simulink model "robotarm_part_both"  (R2018b)
settings: Solver=FixedStepAuto  StartTime=0.0  StopTime=options.T_train-options.dt  RelTol=1e-3  AbsTol=1e-6
undefined symbols (not defined in the file or in its folder): options
libraries: neural x132, simulink x4
(part 4 of 6)

== system robotarm_part_both/NN/Layer 3/Delays 1 ==
  "p{3}" : Inport  PortDimensions=30
      mask Display: e = 0.06;c1 = [120 230 180]/255;c2 = ([120 230 180]+0)/(256+128);c3 = ([120 230 180]+128)/(256+128);patch([0 1 1 0],[0 0 1 1],c1);patch([0 1 1 1-e 1-e 0+e],[0 0 1 1-e 0+e 0+e],c2);patch([0 0 1 1-e 0+e 0+e],[0 1 1 1-e 1-e 0+e],c3);plot([0 1 1 0 0],[0 0 1 1 0]);
  mux : Mux  Inputs=1
      mask Display: e = 0.06;c1 = [120 150 230]/255;c2 = ([120 150 230]+0)/383;c3 = ([120 150 230]+128)/383;patch([0 1 1 0],[0 0 1 1],c1);patch([0 1 1 1-e 1-e 0+e],[0 0 1 1-e 0+e 0+e],c2);patch([0 0 1 1-e 0+e 0+e],[0 1 1 1-e 1-e 0+e],c3);plot([0 1 1 0 0],[0 0 1 1 0]);disp('Mux')
  "pd{3,2}" : Outport
      mask Display: e = 0.06;c1 = [120 230 180]/255;c2 = ([120 230 180]+0)/(256+128);c3 = ([120 230 180]+128)/(256+128);patch([0 1 1 0],[0 0 1 1],c1);patch([0 1 1 1-e 1-e 0+e],[0 0 1 1-e 0+e 0+e],c2);patch([0 0 1 1-e 0+e 0+e],[0 1 1 1-e 1-e 0+e],c3);plot([0 1 1 0 0],[0 0 1 1 0]);
  wires:
  "p{3}"/1 -> mux/1
  mux/1 -> "pd{3,2}"/1

== system robotarm_part_both/NN/Layer 3/LW{3,2} ==
  "ad{3,2}" : Inport  PortDimensions=30
      mask Display: e = 0.06;c1 = [120 230 180]/255;c2 = ([120 230 180]+0)/(256+128);c3 = ([120 230 180]+128)/(256+128);patch([0 1 1 0],[0 0 1 1],c1);patch([0 1 1 1-e 1-e 0+e],[0 0 1 1-e 0+e 0+e],c2);patch([0 0 1 1-e 0+e 0+e],[0 1 1 1-e 1-e 0+e],c3);plot([0 1 1 0 0],[0 0 1 1 0]);
  "IW{3,2}(1,:)'" : Constant  Value=[0.176394547847553762043304459439241327345371246337890625;-0.1116456887869614333919088267066399566829204559326171875;0.58215121397970370775709625377203337848186492919921875;0.7323597745263732416987068063463084399700164794921875;0.283355295459314759920488313582609407603740692138671875;0.77930108203370540564947077655233442783355712890625;-0.28029976793160094050705311019555665552616119384765625;0.469261371288066830853580313487327657639980316162109375;0.292093450290357881105052229031571187078952789306640625;0.449281302149557693059733765039709396660327911376953125;0.386298724431223872155527487848303280770778656005859375;0.0105704306857183523427057281196539406664669513702392578125;-0.20177765854276685786317102611064910888671875;0.05511109655202676982366227775855804793536663055419921875;-0.5391171282818068011266632311162538826465606689453125;-0.41937710733039512689401817624457180500030517578125;-0.258060070180556488939060955090099014341831207275390625;-0.391205760480985542670850918511860072612762451171875;0.1540637115479316088251238170414580963551998138427734375;-0.372538014477659384926511165758711285889148712158203125;-0.7010359337987279726434053372940979897975921630859375;-0.3311213427238712814215659818728454411029815673828125;-0.07789499457458821940480930834382888861000537872314453125;-0.494423699379576142565184682098333723843097686767578125;-0.321664189878497486230202184742665849626064300537109375;-0.1524588096722032937169188926418428309261798858642578125;0.270977785627045497651721461807028390467166900634765625;-0.237034371203050320264793526803259737789630889892578125;-0.4681526216624172231917100361897610127925872802734375;-0.06115859490412589583030467110802419483661651611328125]
      mask Display: e = 0.06;c1 = [120 150 230]/255;c2 = ([120 150 230]+0)/383;c3 = ([120 150 230]+128)/383;patch([0 1 1 0],[0 0 1 1],c1);patch([0 1 1 1-e 1-e 0+e],[0 0 1 1-e 0+e 0+e],c2);patch([0 0 1 1-e 0+e 0+e],[0 1 1 1-e 1-e 0+e],c3);plot([0 1 1 0 0],[0 0 1 1 0]);disp('weights');
  Mux : Mux  Inputs=1
      mask Display: e = 0.06;c1 = [120 150 230]/255;c2 = ([120 150 230]+0)/383;c3 = ([120 150 230]+128)/383;patch([0 1 1 0],[0 0 1 1],c1);patch([0 1 1 1-e 1-e 0+e],[0 0 1 1-e 0+e 0+e],c2);patch([0 0 1 1-e 0+e 0+e],[0 1 1 1-e 1-e 0+e],c3);plot([0 1 1 0 0],[0 0 1 1 0]);disp('Mux');
  dotprod1 : neural/Weight Functions/dotprod
  "lz{3,2}" : Outport
      mask Display: e = 0.06;c1 = [120 230 180]/255;c2 = ([120 230 180]+0)/(256+128);c3 = ([120 230 180]+128)/(256+128);patch([0 1 1 0],[0 0 1 1],c1);patch([0 1 1 1-e 1-e 0+e],[0 0 1 1-e 0+e 0+e],c2);patch([0 0 1 1-e 0+e 0+e],[0 1 1 1-e 1-e 0+e],c3);plot([0 1 1 0 0],[0 0 1 1 0]);
  wires:
  "IW{3,2}(1,:)'"/1 -> dotprod1/1
  "ad{3,2}"/1 -> dotprod1/2
  dotprod1/1 -> Mux/1
  Mux/1 -> "lz{3,2}"/1

== system robotarm_part_both/NN_cex_1/Layer 1/Delays 1 ==
  "p{1}" : Inport  PortDimensions=10
      mask Display: e = 0.06;c1 = [120 230 180]/255;c2 = ([120 230 180]+0)/(256+128);c3 = ([120 230 180]+128)/(256+128);patch([0 1 1 0],[0 0 1 1],c1);patch([0 1 1 1-e 1-e 0+e],[0 0 1 1-e 0+e 0+e],c2);patch([0 0 1 1-e 0+e 0+e],[0 1 1 1-e 1-e 0+e],c3);plot([0 1 1 0 0],[0 0 1 1 0]);
  mux : Mux  Inputs=1
      mask Display: e = 0.06;c1 = [120 150 230]/255;c2 = ([120 150 230]+0)/383;c3 = ([120 150 230]+128)/383;patch([0 1 1 0],[0 0 1 1],c1);patch([0 1 1 1-e 1-e 0+e],[0 0 1 1-e 0+e 0+e],c2);patch([0 0 1 1-e 0+e 0+e],[0 1 1 1-e 1-e 0+e],c3);plot([0 1 1 0 0],[0 0 1 1 0]);disp('Mux')
  "pd{1,1}" : Outport
      mask Display: e = 0.06;c1 = [120 230 180]/255;c2 = ([120 230 180]+0)/(256+128);c3 = ([120 230 180]+128)/(256+128);patch([0 1 1 0],[0 0 1 1],c1);patch([0 1 1 1-e 1-e 0+e],[0 0 1 1-e 0+e 0+e],c2);patch([0 0 1 1-e 0+e 0+e],[0 1 1 1-e 1-e 0+e],c3);plot([0 1 1 0 0],[0 0 1 1 0]);
  wires:
  "p{1}"/1 -> mux/1
  mux/1 -> "pd{1,1}"/1

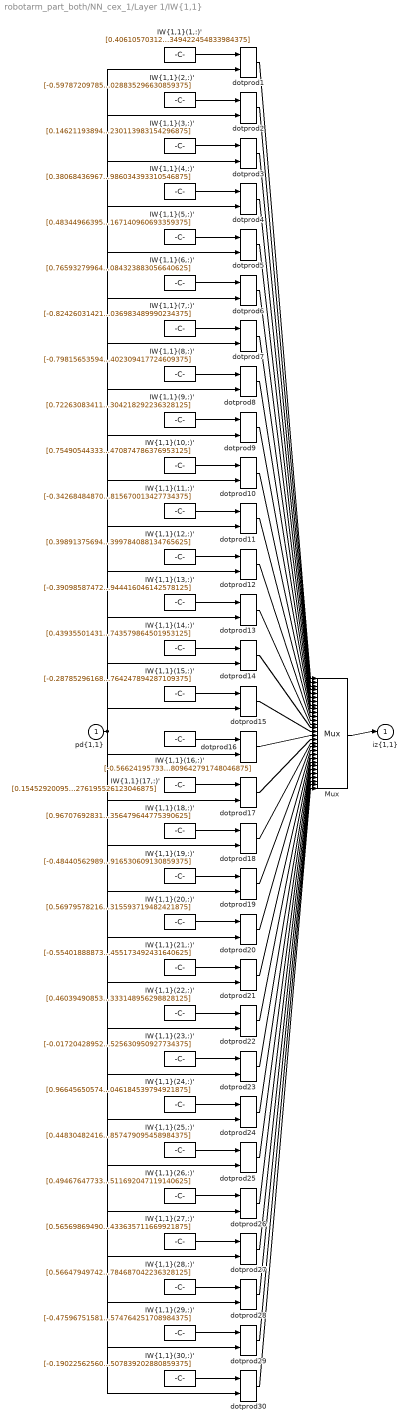
== system robotarm_part_both/NN_cex_1/Layer 1/IW{1,1} ==
  "pd{1,1}" : Inport  PortDimensions=10
      mask Display: e = 0.06;c1 = [120 230 180]/255;c2 = ([120 230 180]+0)/(256+128);c3 = ([120 230 180]+128)/(256+128);patch([0 1 1 0],[0 0 1 1],c1);patch([0 1 1 1-e 1-e 0+e],[0 0 1 1-e 0+e 0+e],c2);patch([0 0 1 1-e 0+e 0+e],[0 1 1 1-e 1-e 0+e],c3);plot([0 1 1 0 0],[0 0 1 1 0]);
  "IW{1,1}(1,:)'" : Constant  Value=[0.40610570312081251120872593673993833363056182861328125;-0.0618337729401200186796216939910664223134517669677734375;-0.027542948468563401009934210605933913029730319976806640625;-0.74658296364276865997311460887431167066097259521484375;0.0647152481491918563083487470066756941378116607666015625;0.532009309863485935210292154806666076183319091796875;-0.051795183452861430495328676215649466030299663543701171875;1.16180416143057296807228340185247361660003662109375;0.403930434889277767407378405550844036042690277099609375;-0.70819180118117885935902222627191804349422454833984375]
      mask Display: e = 0.06;c1 = [120 150 230]/255;c2 = ([120 150 230]+0)/383;c3 = ([120 150 230]+128)/383;patch([0 1 1 0],[0 0 1 1],c1);patch([0 1 1 1-e 1-e 0+e],[0 0 1 1-e 0+e 0+e],c2);patch([0 0 1 1-e 0+e 0+e],[0 1 1 1-e 1-e 0+e],c3);plot([0 1 1 0 0],[0 0 1 1 0]);disp('Weights');
  "IW{1,1}(10,:)'" : Constant  Value=[0.754905443337720694074732818990014493465423583984375;-0.2307145756276104131554660625624819658696651458740234375;-0.058374557330017916301212466123615740798413753509521484375;0.80634010994632199231801905625616200268268585205078125;-0.387179161003805616392270394499064423143863677978515625;0.4883646797805132333536448641098104417324066162109375;0.9334065215820845917704673411208204925060272216796875;-0.68294902726114614655017476252396591007709503173828125;0.57946714263174925463317777030169963836669921875;-0.384973810509336378249400922868517227470874786376953125]
      mask Display: e = 0.06;c1 = [120 150 230]/255;c2 = ([120 150 230]+0)/383;c3 = ([120 150 230]+128)/383;patch([0 1 1 0],[0 0 1 1],c1);patch([0 1 1 1-e 1-e 0+e],[0 0 1 1-e 0+e 0+e],c2);patch([0 0 1 1-e 0+e 0+e],[0 1 1 1-e 1-e 0+e],c3);plot([0 1 1 0 0],[0 0 1 1 0]);disp('Weights');
  "IW{1,1}(11,:)'" : Constant  Value=[-0.342684848708500300329404808508115820586681365966796875;-0.4011699929023067046074402242084033787250518798828125;1.0598889739814121302430294235819019377231597900390625;-0.2566824900326813985174112531240098178386688232421875;0.286617566677122737051064405022771097719669342041015625;0.437452894939382719297071844266611151397228240966796875;-0.83506440735054210389165518790832720696926116943359375;0.281658478227369057922402362237335182726383209228515625;0.47340709091096166982737258877023123204708099365234375;0.98784426306218531266267746104858815670013427734375]
      mask Display: e = 0.06;c1 = [120 150 230]/255;c2 = ([120 150 230]+0)/383;c3 = ([120 150 230]+128)/383;patch([0 1 1 0],[0 0 1 1],c1);patch([0 1 1 1-e 1-e 0+e],[0 0 1 1-e 0+e 0+e],c2);patch([0 0 1 1-e 0+e 0+e],[0 1 1 1-e 1-e 0+e],c3);plot([0 1 1 0 0],[0 0 1 1 0]);disp('Weights');
  "IW{1,1}(12,:)'" : Constant  Value=[0.398913756949194342471542995554045774042606353759765625;-1.0219642473780263802751733237528242170810699462890625;0.66452831996743022546780821357970125973224639892578125;0.7230875011438542276920315998722799122333526611328125;0.06718552543198720583550453966381610371172428131103515625;0.25328258897489164258587379663367755711078643798828125;0.04377790583161665638467496819430380128324031829833984375;0.2465544725107126355911901782747008837759494781494140625;0.380746784031783802593196242014528252184391021728515625;0.698639278926427298443968538776971399784088134765625]
      mask Display: e = 0.06;c1 = [120 150 230]/255;c2 = ([120 150 230]+0)/383;c3 = ([120 150 230]+128)/383;patch([0 1 1 0],[0 0 1 1],c1);patch([0 1 1 1-e 1-e 0+e],[0 0 1 1-e 0+e 0+e],c2);patch([0 0 1 1-e 0+e 0+e],[0 1 1 1-e 1-e 0+e],c3);plot([0 1 1 0 0],[0 0 1 1 0]);disp('Weights');
  "IW{1,1}(13,:)'" : Constant  Value=[-0.390985874725247761762858544898335821926593780517578125;0.68715563779107657893518990022130310535430908203125;-0.05459024117889653415769402045043534599244594573974609375;0.493818674941325530536317955920821987092494964599609375;0.93328497180974079316939651107531972229480743408203125;-0.04136663725988042050740745025905198417603969573974609375;0.51698619349367913589077261349302716553211212158203125;-0.2237583707189104986756689186222502030432224273681640625;0.63723107769787101783975913349422626197338104248046875;-0.888813604233327669845721175079233944416046142578125]
      mask Display: e = 0.06;c1 = [120 150 230]/255;c2 = ([120 150 230]+0)/383;c3 = ([120 150 230]+128)/383;patch([0 1 1 0],[0 0 1 1],c1);patch([0 1 1 1-e 1-e 0+e],[0 0 1 1-e 0+e 0+e],c2);patch([0 0 1 1-e 0+e 0+e],[0 1 1 1-e 1-e 0+e],c3);plot([0 1 1 0 0],[0 0 1 1 0]);disp('Weights');
  "IW{1,1}(14,:)'" : Constant  Value=[0.439355014317911740651112495470442809164524078369140625;-0.6120670869240980582759448225260712206363677978515625;-0.80865955894022889527406050547142513096332550048828125;0.371840320627411846654553073676652275025844573974609375;-0.94104647756993109464218605353380553424358367919921875;1.0656100492619675623728880964335985481739044189453125;0.215787684182779881947311650947085581719875335693359375;0.305366971574978440795433698440319858491420745849609375;-0.03747921878648863280858449797960929572582244873046875;0.114143621883545709483342989187804050743579864501953125]
      mask Display: e = 0.06;c1 = [120 150 230]/255;c2 = ([120 150 230]+0)/383;c3 = ([120 150 230]+128)/383;patch([0 1 1 0],[0 0 1 1],c1);patch([0 1 1 1-e 1-e 0+e],[0 0 1 1-e 0+e 0+e],c2);patch([0 0 1 1-e 0+e 0+e],[0 1 1 1-e 1-e 0+e],c3);plot([0 1 1 0 0],[0 0 1 1 0]);disp('Weights');
  "IW{1,1}(15,:)'" : Constant  Value=[-0.287852961686321240364350160234607756137847900390625;0.193811697275944105900435943112825043499469757080078125;-0.8410307478423624250041257255361415445804595947265625;0.84437904998481816409849898263928480446338653564453125;0.29952993297291474750210227284696884453296661376953125;0.27291419885216672280847660658764652907848358154296875;0.6419725776834723784958214309881441295146942138671875;-0.10748546258155665389377730889464146457612514495849609375;-0.478464668092987377434610607451759278774261474609375;-0.6291180402851974662326028919778764247894287109375]
      mask Display: e = 0.06;c1 = [120 150 230]/255;c2 = ([120 150 230]+0)/383;c3 = ([120 150 230]+128)/383;patch([0 1 1 0],[0 0 1 1],c1);patch([0 1 1 1-e 1-e 0+e],[0 0 1 1-e 0+e 0+e],c2);patch([0 0 1 1-e 0+e 0+e],[0 1 1 1-e 1-e 0+e],c3);plot([0 1 1 0 0],[0 0 1 1 0]);disp('Weights');
  "IW{1,1}(16,:)'" : Constant  Value=[-0.5662419573309234177571624968550167977809906005859375;0.504981057654423803882082211202941834926605224609375;-1.1343989356561134940193369402550160884857177734375;-0.075054956664876215644000012616743333637714385986328125;-0.85555149227211002571635845015407539904117584228515625;-0.189969480968393444886288534689811058342456817626953125;0.257703553768643456312048556355875916779041290283203125;-0.114101898538623292012061938294209539890289306640625;-0.01034982455533548471870997076393905445002019405364990234375;-0.03712863475843779237361985678944620303809642791748046875]
      mask Display: e = 0.06;c1 = [120 150 230]/255;c2 = ([120 150 230]+0)/383;c3 = ([120 150 230]+128)/383;patch([0 1 1 0],[0 0 1 1],c1);patch([0 1 1 1-e 1-e 0+e],[0 0 1 1-e 0+e 0+e],c2);patch([0 0 1 1-e 0+e 0+e],[0 1 1 1-e 1-e 0+e],c3);plot([0 1 1 0 0],[0 0 1 1 0]);disp('Weights');
  "IW{1,1}(17,:)'" : Constant  Value=[0.154529200951685208309527297387830913066864013671875;0.48354369097717586623019769831444136798381805419921875;0.692335704444002164592575354618020355701446533203125;0.33065881691269505271435491522424854338169097900390625;0.700715460652138855124348992831073701381683349609375;0.9392393355523533937656566195073537528514862060546875;-0.83768647200012946729685836544376797974109649658203125;-0.278233473644368178856467466175672598183155059814453125;0.375486157959734168088061778689734637737274169921875;0.11365059515114765698040599772866698913276195526123046875]
      mask Display: e = 0.06;c1 = [120 150 230]/255;c2 = ([120 150 230]+0)/383;c3 = ([120 150 230]+128)/383;patch([0 1 1 0],[0 0 1 1],c1);patch([0 1 1 1-e 1-e 0+e],[0 0 1 1-e 0+e 0+e],c2);patch([0 0 1 1-e 0+e 0+e],[0 1 1 1-e 1-e 0+e],c3);plot([0 1 1 0 0],[0 0 1 1 0]);disp('Weights');
  "IW{1,1}(18,:)'" : Constant  Value=[0.967076928319382300713868971797637641429901123046875;-0.66164947528674133980786109532346017658710479736328125;-0.3141703919957035129328914990765042603015899658203125;-0.93982557986142711836663465874153189361095428466796875;-0.5448594698446898032528906696825288236141204833984375;0.1274965495680859539628926313525880686938762664794921875;0.403484102726418936146757232563686557114124298095703125;-0.450081409216426531205712535665952600538730621337890625;0.404013712675034331045509361501899547874927520751953125;0.69614128919235407355614597690873779356479644775390625]
      mask Display: e = 0.06;c1 = [120 150 230]/255;c2 = ([120 150 230]+0)/383;c3 = ([120 150 230]+128)/383;patch([0 1 1 0],[0 0 1 1],c1);patch([0 1 1 1-e 1-e 0+e],[0 0 1 1-e 0+e 0+e],c2);patch([0 0 1 1-e 0+e 0+e],[0 1 1 1-e 1-e 0+e],c3);plot([0 1 1 0 0],[0 0 1 1 0]);disp('Weights');
  "IW{1,1}(19,:)'" : Constant  Value=[-0.484405629893030875710024929503560997545719146728515625;0.77945971793746637867883464423357509076595306396484375;-0.278649568567306105126846205166657455265522003173828125;0.49799572768193989258378451268072240054607391357421875;-0.388289522122739760856546809009159915149211883544921875;0.162724212432617532098078072522184811532497406005859375;0.764539980173248867600932499044574797153472900390625;-0.6912157507333909212121625387226231396198272705078125;-0.9166608172565313683577414849423803389072418212890625;-0.7061016716226686806834322851500473916530609130859375]
      mask Display: e = 0.06;c1 = [120 150 230]/255;c2 = ([120 150 230]+0)/383;c3 = ([120 150 230]+128)/383;patch([0 1 1 0],[0 0 1 1],c1);patch([0 1 1 1-e 1-e 0+e],[0 0 1 1-e 0+e 0+e],c2);patch([0 0 1 1-e 0+e 0+e],[0 1 1 1-e 1-e 0+e],c3);plot([0 1 1 0 0],[0 0 1 1 0]);disp('Weights');
  "IW{1,1}(2,:)'" : Constant  Value=[-0.5978720978507292560522046187543310225009918212890625;-0.451225889460342977077544901476358063519001007080078125;0.73115114985429396909921706537716090679168701171875;-0.33177832418549713100475173632730729877948760986328125;0.5656634448348001331652312728692777454853057861328125;0.203845531538278501582084345500334165990352630615234375;0.60328541488133613501787522181984968483448028564453125;-0.295759245605732079553717994713224470615386962890625;-0.863527859816612508581101792515255510807037353515625;-0.8686108953587632353077196967205964028835296630859375]
      mask Display: e = 0.06;c1 = [120 150 230]/255;c2 = ([120 150 230]+0)/383;c3 = ([120 150 230]+128)/383;patch([0 1 1 0],[0 0 1 1],c1);patch([0 1 1 1-e 1-e 0+e],[0 0 1 1-e 0+e 0+e],c2);patch([0 0 1 1-e 0+e 0+e],[0 1 1 1-e 1-e 0+e],c3);plot([0 1 1 0 0],[0 0 1 1 0]);disp('Weights');
  "IW{1,1}(20,:)'" : Constant  Value=[0.569795782163188935243169908062554895877838134765625;-0.175366068818801290607467535664909519255161285400390625;0.299468569242130888685693435036228038370609283447265625;0.00013019514896176246319947633622859939350746572017669677734375;-0.913508827616769547574904208886437118053436279296875;1.2317060303614313365727639393298886716365814208984375;-0.310041832148403584401563648498267866671085357666015625;-0.68644604330826031191037372991559095680713653564453125;-0.02734988959488722504165281179666635580360889434814453125;-0.1646195679784154541902552182364161126315593719482421875]
      mask Display: e = 0.06;c1 = [120 150 230]/255;c2 = ([120 150 230]+0)/383;c3 = ([120 150 230]+128)/383;patch([0 1 1 0],[0 0 1 1],c1);patch([0 1 1 1-e 1-e 0+e],[0 0 1 1-e 0+e 0+e],c2);patch([0 0 1 1-e 0+e 0+e],[0 1 1 1-e 1-e 0+e],c3);plot([0 1 1 0 0],[0 0 1 1 0]);disp('Weights');
  "IW{1,1}(21,:)'" : Constant  Value=[-0.554018888738172510244339719065465033054351806640625;-0.428769524213964914327590349785168655216693878173828125;-0.0800834615707680941287804898820468224585056304931640625;-0.8169714872980133879565300958347506821155548095703125;-0.6459854934693691763669676220160908997058868408203125;0.58988824050972965551409288309514522552490234375;0.2646341908830576183930816114298067986965179443359375;-0.68226497917992612318727196907275356352329254150390625;0.389913364883176460917724170940346084535121917724609375;0.671389074260846374642142109223641455173492431640625]
      mask Display: e = 0.06;c1 = [120 150 230]/255;c2 = ([120 150 230]+0)/383;c3 = ([120 150 230]+128)/383;patch([0 1 1 0],[0 0 1 1],c1);patch([0 1 1 1-e 1-e 0+e],[0 0 1 1-e 0+e 0+e],c2);patch([0 0 1 1-e 0+e 0+e],[0 1 1 1-e 1-e 0+e],c3);plot([0 1 1 0 0],[0 0 1 1 0]);disp('Weights');
  "IW{1,1}(22,:)'" : Constant  Value=[0.460394908538499125771892295233556069433689117431640625;0.69299410430707297781083298104931600391864776611328125;-0.58147459969207215824127388259512372314929962158203125;-0.474008418395088726438046933253644965589046478271484375;-0.19586296063152819346697697255876846611499786376953125;-0.5774582392745102321640615627984516322612762451171875;0.915756888185493611587162376963533461093902587890625;-0.844006379670238171541996052837930619716644287109375;-0.62517377429491582940812577362521551549434661865234375;-0.394218307905169595972694196461816318333148956298828125]
      mask Display: e = 0.06;c1 = [120 150 230]/255;c2 = ([120 150 230]+0)/383;c3 = ([120 150 230]+128)/383;patch([0 1 1 0],[0 0 1 1],c1);patch([0 1 1 1-e 1-e 0+e],[0 0 1 1-e 0+e 0+e],c2);patch([0 0 1 1-e 0+e 0+e],[0 1 1 1-e 1-e 0+e],c3);plot([0 1 1 0 0],[0 0 1 1 0]);disp('Weights');
  "IW{1,1}(23,:)'" : Constant  Value=[-0.01720428952464754523976608879820560105144977569580078125;0.0915619286382170771698696398743777535855770111083984375;-0.216310552483802209788876780294231139123439788818359375;0.683699817299082912569474501651711761951446533203125;0.55572107062446374214914612821303308010101318359375;-0.38831201307937046607321462943218648433685302734375;0.74460998939169098509438526889425702393054962158203125;-0.412168552568078883080460173005121760070323944091796875;0.296429067542405111357339819733169861137866973876953125;-0.903105169254780459908715783967636525630950927734375]
      mask Display: e = 0.06;c1 = [120 150 230]/255;c2 = ([120 150 230]+0)/383;c3 = ([120 150 230]+128)/383;patch([0 1 1 0],[0 0 1 1],c1);patch([0 1 1 1-e 1-e 0+e],[0 0 1 1-e 0+e 0+e],c2);patch([0 0 1 1-e 0+e 0+e],[0 1 1 1-e 1-e 0+e],c3);plot([0 1 1 0 0],[0 0 1 1 0]);disp('Weights');
  "IW{1,1}(24,:)'" : Constant  Value=[0.9664565057440073214678477597772143781185150146484375;0.08297129843086743783420189402022515423595905303955078125;-0.782415106607832644414202150073833763599395751953125;-0.62027706726544362680897393147461116313934326171875;0.7418119761811379220262097078375518321990966796875;-0.7912576799074060307503941658069379627704620361328125;0.15814280110847656057870835866197012364864349365234375;-0.47819226762323463475468088290654122829437255859375;0.44516983178018654232488415800617076456546783447265625;-0.1378403995316616892363725810355390422046184539794921875]
      mask Display: e = 0.06;c1 = [120 150 230]/255;c2 = ([120 150 230]+0)/383;c3 = ([120 150 230]+128)/383;patch([0 1 1 0],[0 0 1 1],c1);patch([0 1 1 1-e 1-e 0+e],[0 0 1 1-e 0+e 0+e],c2);patch([0 0 1 1-e 0+e 0+e],[0 1 1 1-e 1-e 0+e],c3);plot([0 1 1 0 0],[0 0 1 1 0]);disp('Weights');
  "IW{1,1}(25,:)'" : Constant  Value=[0.448304824162995718683788481939700432121753692626953125;-0.441083545672387666858327293084585107862949371337890625;-0.7086421050067974736208498143241740763187408447265625;0.805571336795230852345639505074359476566314697265625;0.7757330590206288345456187016679905354976654052734375;-0.258695728383482370649204540313803590834140777587890625;-0.40794372310651982882490074189263395965099334716796875;0.264501362790562855042963974483427591621875762939453125;0.56836095891894611309425044964882545173168182373046875;0.94902066957128194957249434082768857479095458984375]
      mask Display: e = 0.06;c1 = [120 150 230]/255;c2 = ([120 150 230]+0)/383;c3 = ([120 150 230]+128)/383;patch([0 1 1 0],[0 0 1 1],c1);patch([0 1 1 1-e 1-e 0+e],[0 0 1 1-e 0+e 0+e],c2);patch([0 0 1 1-e 0+e 0+e],[0 1 1 1-e 1-e 0+e],c3);plot([0 1 1 0 0],[0 0 1 1 0]);disp('Weights');
  "IW{1,1}(26,:)'" : Constant  Value=[0.494676477332296193889504820617730729281902313232421875;-0.51418734519718201081417419118224643170833587646484375;-0.53269214219483107530805909846094436943531036376953125;-0.326399857319428277069306432167650200426578521728515625;-0.641083256409577639800545512116514146327972412109375;-0.661372013967330030226321468944661319255828857421875;-0.51378225686084999512814874833566136658191680908203125;-0.7031859535346625111884577563614584505558013916015625;0.71167339493647296944089930548216216266155242919921875;-0.253121486450810895263430211343802511692047119140625]
      mask Display: e = 0.06;c1 = [120 150 230]/255;c2 = ([120 150 230]+0)/383;c3 = ([120 150 230]+128)/383;patch([0 1 1 0],[0 0 1 1],c1);patch([0 1 1 1-e 1-e 0+e],[0 0 1 1-e 0+e 0+e],c2);patch([0 0 1 1-e 0+e 0+e],[0 1 1 1-e 1-e 0+e],c3);plot([0 1 1 0 0],[0 0 1 1 0]);disp('Weights');
  "IW{1,1}(27,:)'" : Constant  Value=[0.56569869490757884733511673402972519397735595703125;0.55932485469986747972370721981860697269439697265625;0.757553169851645780141780051053501665592193603515625;0.445739884859973678477018665944342501461505889892578125;-0.052810541890100599904389611083388444967567920684814453125;-0.5124647759251439449457166119827888906002044677734375;0.1453672125440539086849156547032180242240428924560546875;0.5844524834818864977847852060222066938877105712890625;0.301678561512196796723372926862793974578380584716796875;0.67239156025882074185773262797738425433635711669921875]
      mask Display: e = 0.06;c1 = [120 150 230]/255;c2 = ([120 150 230]+0)/383;c3 = ([120 150 230]+128)/383;patch([0 1 1 0],[0 0 1 1],c1);patch([0 1 1 1-e 1-e 0+e],[0 0 1 1-e 0+e 0+e],c2);patch([0 0 1 1-e 0+e 0+e],[0 1 1 1-e 1-e 0+e],c3);plot([0 1 1 0 0],[0 0 1 1 0]);disp('Weights');
  "IW{1,1}(28,:)'" : Constant  Value=[0.56647949742772751857700086475233547389507293701171875;-0.6072031078302975171112620955682359635829925537109375;-0.0252895405359683279888916018762756721116602420806884765625;-0.59420130639994450660879010683856904506683349609375;-0.8370146046590443145163362714811228215694427490234375;-0.2168133856068210629786108256666921079158782958984375;-0.0278184788230993497448739759647651226259768009185791015625;0.170700644385492206200893861023359932005405426025390625;-0.89753992568694818121599610094563104212284088134765625;-0.88615362909724126883048711533774621784687042236328125]
      mask Display: e = 0.06;c1 = [120 150 230]/255;c2 = ([120 150 230]+0)/383;c3 = ([120 150 230]+128)/383;patch([0 1 1 0],[0 0 1 1],c1);patch([0 1 1 1-e 1-e 0+e],[0 0 1 1-e 0+e 0+e],c2);patch([0 0 1 1-e 0+e 0+e],[0 1 1 1-e 1-e 0+e],c3);plot([0 1 1 0 0],[0 0 1 1 0]);disp('Weights');
  "IW{1,1}(29,:)'" : Constant  Value=[-0.47596751581870855307698775504832156002521514892578125;0.61043374535515082524028684929362498223781585693359375;0.6728816456322224137664989029872231185436248779296875;0.486894561880593490510449328212416730821132659912109375;0.61933355086790087273840299531002528965473175048828125;-0.457033928935499600409997356109670363366603851318359375;-0.66696973339012910475531725751352496445178985595703125;-0.5293927524224042446832072528195567429065704345703125;0.0993688407071657009428378160009742714464664459228515625;0.8282155411331133532115700290887616574764251708984375]
      mask Display: e = 0.06;c1 = [120 150 230]/255;c2 = ([120 150 230]+0)/383;c3 = ([120 150 230]+128)/383;patch([0 1 1 0],[0 0 1 1],c1);patch([0 1 1 1-e 1-e 0+e],[0 0 1 1-e 0+e 0+e],c2);patch([0 0 1 1-e 0+e 0+e],[0 1 1 1-e 1-e 0+e],c3);plot([0 1 1 0 0],[0 0 1 1 0]);disp('Weights');
  "IW{1,1}(3,:)'" : Constant  Value=[0.1462119389481443543221672598519944585859775543212890625;0.5409826763721661269102014557574875652790069580078125;-0.5796650085556314113688358702347613871097564697265625;-0.30474880936511306028791068456484936177730560302734375;0.564453778928731164654664098634384572505950927734375;-0.81205952454796881401222208296530880033969879150390625;0.69214898994410345434147302512428723275661468505859375;0.6128636765273076658644413328147493302822113037109375;-0.158138791240949594385512000371818430721759796142578125;-0.79754389040653339559838741479325108230113983154296875]
      mask Display: e = 0.06;c1 = [120 150 230]/255;c2 = ([120 150 230]+0)/383;c3 = ([120 150 230]+128)/383;patch([0 1 1 0],[0 0 1 1],c1);patch([0 1 1 1-e 1-e 0+e],[0 0 1 1-e 0+e 0+e],c2);patch([0 0 1 1-e 0+e 0+e],[0 1 1 1-e 1-e 0+e],c3);plot([0 1 1 0 0],[0 0 1 1 0]);disp('Weights');
  "IW{1,1}(30,:)'" : Constant  Value=[-0.190225625600574044238300075448933057487010955810546875;0.017468262158388904448091949461741023696959018707275390625;-0.6132260054544051985914165925350971519947052001953125;-0.82029990501021987636676158217596821486949920654296875;-0.1386236818221863453803877064274274744093418121337890625;-0.829748698933009176670339002157561480998992919921875;-0.8670919641264187571749744165572337806224822998046875;0.199950952276734372770050640610861591994762420654296875;0.311014114925649121090600601746700704097747802734375;-0.02855041527662149913879829910001717507839202880859375]
      mask Display: e = 0.06;c1 = [120 150 230]/255;c2 = ([120 150 230]+0)/383;c3 = ([120 150 230]+128)/383;patch([0 1 1 0],[0 0 1 1],c1);patch([0 1 1 1-e 1-e 0+e],[0 0 1 1-e 0+e 0+e],c2);patch([0 0 1 1-e 0+e 0+e],[0 1 1 1-e 1-e 0+e],c3);plot([0 1 1 0 0],[0 0 1 1 0]);disp('Weights');
  "IW{1,1}(4,:)'" : Constant  Value=[0.38068436967307361928902764702797867357730865478515625;0.28417303818815697891153604359715245664119720458984375;0.7312009406319954774033931244048289954662322998046875;-0.024292985054512071518839633199604577384889125823974609375;0.84976082856418144739762965400586836040019989013671875;0.59084861804597021972540460410527884960174560546875;-0.0925035231488953446632450550168869085609912872314453125;0.665146318220788401731624617241322994232177734375;-0.6326178942232971724735079988022334873676300048828125;0.4876558849691245978164033658686093986034393310546875]
      mask Display: e = 0.06;c1 = [120 150 230]/255;c2 = ([120 150 230]+0)/383;c3 = ([120 150 230]+128)/383;patch([0 1 1 0],[0 0 1 1],c1);patch([0 1 1 1-e 1-e 0+e],[0 0 1 1-e 0+e 0+e],c2);patch([0 0 1 1-e 0+e 0+e],[0 1 1 1-e 1-e 0+e],c3);plot([0 1 1 0 0],[0 0 1 1 0]);disp('Weights');
  "IW{1,1}(5,:)'" : Constant  Value=[0.483449663950935637490857743614469654858112335205078125;0.59182958335229252089249030177597887814044952392578125;-1.019668457319926613280358651536516845226287841796875;0.1601651360603670026794276282089413143694400787353515625;0.513959511416858472188096129684709012508392333984375;0.41566689975038750848312929520034231245517730712890625;-0.09983684809643979252147261149730184115469455718994140625;-0.95413479169471770990895720387925393879413604736328125;0.65426938387890720694173296578810550272464752197265625;-0.0676400009371243837730247605577460490167140960693359375]
      mask Display: e = 0.06;c1 = [120 150 230]/255;c2 = ([120 150 230]+0)/383;c3 = ([120 150 230]+128)/383;patch([0 1 1 0],[0 0 1 1],c1);patch([0 1 1 1-e 1-e 0+e],[0 0 1 1-e 0+e 0+e],c2);patch([0 0 1 1-e 0+e 0+e],[0 1 1 1-e 1-e 0+e],c3);plot([0 1 1 0 0],[0 0 1 1 0]);disp('Weights');
  "IW{1,1}(6,:)'" : Constant  Value=[0.7659327996434068808184747467748820781707763671875;0.1209203413188399967026498416089452803134918212890625;-0.2011201291618239517244859371203347109258174896240234375;-1.0085378395964486042402086241054348647594451904296875;-0.755905735818904300771237103617750108242034912109375;0.21109003195339448577527718953206203877925872802734375;-0.567068725201946843839095890871249139308929443359375;0.96488706863451556561273037004866637289524078369140625;-0.1600338643666720794822566631410154514014720916748046875;-0.166087200947841184817121984451659955084323883056640625]
      mask Display: e = 0.06;c1 = [120 150 230]/255;c2 = ([120 150 230]+0)/383;c3 = ([120 150 230]+128)/383;patch([0 1 1 0],[0 0 1 1],c1);patch([0 1 1 1-e 1-e 0+e],[0 0 1 1-e 0+e 0+e],c2);patch([0 0 1 1-e 0+e 0+e],[0 1 1 1-e 1-e 0+e],c3);plot([0 1 1 0 0],[0 0 1 1 0]);disp('Weights');
  "IW{1,1}(7,:)'" : Constant  Value=[-0.8242603142133140270431113094673492014408111572265625;0.000807387174731619594765519298817935123224742710590362548828125;0.6669815484979404462961838362389244139194488525390625;0.155388800449773711864764891288359649479389190673828125;0.018351376132609786839822163528879173099994659423828125;-0.96955498378064408626642034505493938922882080078125;0.72180731663802399911133989007794298231601715087890625;-0.103136383230038319869237284365226514637470245361328125;-0.30727604301804856135049703880213201045989990234375;-0.940873888284963211248168590827845036983489990234375]
      mask Display: e = 0.06;c1 = [120 150 230]/255;c2 = ([120 150 230]+0)/383;c3 = ([120 150 230]+128)/383;patch([0 1 1 0],[0 0 1 1],c1);patch([0 1 1 1-e 1-e 0+e],[0 0 1 1-e 0+e 0+e],c2);patch([0 0 1 1-e 0+e 0+e],[0 1 1 1-e 1-e 0+e],c3);plot([0 1 1 0 0],[0 0 1 1 0]);disp('Weights');
  "IW{1,1}(8,:)'" : Constant  Value=[-0.79815653594790381131218737209565006196498870849609375;1.168230660860092751107686126488260924816131591796875;0.212506187263820034427652672093245200812816619873046875;-0.1983613971877739856619626834799419157207012176513671875;0.358860574747935257011732801402104087173938751220703125;-0.67275296149234831144525514901033602654933929443359375;0.06015785259916250904410617295070551335811614990234375;0.09407483090144251602904290621154359541833400726318359375;1.0988044210287266633230274237575940787792205810546875;0.08409258346176817777717360513634048402309417724609375]
      mask Display: e = 0.06;c1 = [120 150 230]/255;c2 = ([120 150 230]+0)/383;c3 = ([120 150 230]+128)/383;patch([0 1 1 0],[0 0 1 1],c1);patch([0 1 1 1-e 1-e 0+e],[0 0 1 1-e 0+e 0+e],c2);patch([0 0 1 1-e 0+e 0+e],[0 1 1 1-e 1-e 0+e],c3);plot([0 1 1 0 0],[0 0 1 1 0]);disp('Weights');
  "IW{1,1}(9,:)'" : Constant  Value=[0.72263083411855888460451069477130658924579620361328125;-0.84246443815303617697054505697451531887054443359375;0.0172219742555121506366599959392260643653571605682373046875;-0.11925307708007372442526872191592701710760593414306640625;-0.368730549876505830919626305330893956124782562255859375;-0.25418420588322632180933169365744106471538543701171875;0.858428519019280855673059704713523387908935546875;-0.420025547429507317698238466618931852281093597412109375;-0.60283998026069751663413853748352266848087310791015625;-0.561374365570600719621552343596704304218292236328125]
      mask Display: e = 0.06;c1 = [120 150 230]/255;c2 = ([120 150 230]+0)/383;c3 = ([120 150 230]+128)/383;patch([0 1 1 0],[0 0 1 1],c1);patch([0 1 1 1-e 1-e 0+e],[0 0 1 1-e 0+e 0+e],c2);patch([0 0 1 1-e 0+e 0+e],[0 1 1 1-e 1-e 0+e],c3);plot([0 1 1 0 0],[0 0 1 1 0]);disp('Weights');
  Mux : Mux  Inputs=30
      mask Display: e = 0.06;c1 = [120 150 230]/255;c2 = ([120 150 230]+0)/383;c3 = ([120 150 230]+128)/383;patch([0 1 1 0],[0 0 1 1],c1);patch([0 1 1 1-e 1-e 0+e],[0 0 1 1-e 0+e 0+e],c2);patch([0 0 1 1-e 0+e 0+e],[0 1 1 1-e 1-e 0+e],c3);plot([0 1 1 0 0],[0 0 1 1 0]);disp('Mux');
  dotprod{1..30} (30 alike) : neural/Weight Functions/dotprod
  "iz{1,1}" : Outport
      mask Display: e = 0.06;c1 = [120 230 180]/255;c2 = ([120 230 180]+0)/(256+128);c3 = ([120 230 180]+128)/(256+128);patch([0 1 1 0],[0 0 1 1],c1);patch([0 1 1 1-e 1-e 0+e],[0 0 1 1-e 0+e 0+e],c2);patch([0 0 1 1-e 0+e 0+e],[0 1 1 1-e 1-e 0+e],c3);plot([0 1 1 0 0],[0 0 1 1 0]);
  wires:
  "IW{1,1}(1,:)'"/1 -> dotprod1/1
  "pd{1,1}"/1 -> dotprod1/2, dotprod2/2, dotprod3/2, dotprod4/2, dotprod5/2, dotprod6/2, dotprod7/2, dotprod8/2, dotprod9/2, dotprod10/2, dotprod11/2, dotprod12/2, dotprod13/2, dotprod14/2, dotprod15/2, dotprod16/2, dotprod17/2, dotprod18/2, dotprod19/2, dotprod20/2, dotprod21/2, dotprod22/2, dotprod23/2, dotprod24/2, dotprod25/2, dotprod26/2, dotprod27/2, dotprod28/2, dotprod29/2, dotprod30/2
  dotprod1/1 -> Mux/1
  "IW{1,1}(2,:)'"/1 -> dotprod2/1
  dotprod2/1 -> Mux/2
  "IW{1,1}(3,:)'"/1 -> dotprod3/1
  dotprod3/1 -> Mux/3
  "IW{1,1}(4,:)'"/1 -> dotprod4/1
  dotprod4/1 -> Mux/4
  "IW{1,1}(5,:)'"/1 -> dotprod5/1
  dotprod5/1 -> Mux/5
  "IW{1,1}(6,:)'"/1 -> dotprod6/1
  dotprod6/1 -> Mux/6
  "IW{1,1}(7,:)'"/1 -> dotprod7/1
  dotprod7/1 -> Mux/7
  "IW{1,1}(8,:)'"/1 -> dotprod8/1
  dotprod8/1 -> Mux/8
  "IW{1,1}(9,:)'"/1 -> dotprod9/1
  dotprod9/1 -> Mux/9
  "IW{1,1}(10,:)'"/1 -> dotprod10/1
  dotprod10/1 -> Mux/10
  "IW{1,1}(11,:)'"/1 -> dotprod11/1
  dotprod11/1 -> Mux/11
  "IW{1,1}(12,:)'"/1 -> dotprod12/1
  dotprod12/1 -> Mux/12
  "IW{1,1}(13,:)'"/1 -> dotprod13/1
  dotprod13/1 -> Mux/13
  "IW{1,1}(14,:)'"/1 -> dotprod14/1
  dotprod14/1 -> Mux/14
  "IW{1,1}(15,:)'"/1 -> dotprod15/1
  dotprod15/1 -> Mux/15
  "IW{1,1}(16,:)'"/1 -> dotprod16/1
  dotprod16/1 -> Mux/16
  "IW{1,1}(17,:)'"/1 -> dotprod17/1
  dotprod17/1 -> Mux/17
  "IW{1,1}(18,:)'"/1 -> dotprod18/1
  dotprod18/1 -> Mux/18
  "IW{1,1}(19,:)'"/1 -> dotprod19/1
  dotprod19/1 -> Mux/19
  "IW{1,1}(20,:)'"/1 -> dotprod20/1
  dotprod20/1 -> Mux/20
  "IW{1,1}(21,:)'"/1 -> dotprod21/1
  dotprod21/1 -> Mux/21
  "IW{1,1}(22,:)'"/1 -> dotprod22/1
  dotprod22/1 -> Mux/22
  "IW{1,1}(23,:)'"/1 -> dotprod23/1
  dotprod23/1 -> Mux/23
  "IW{1,1}(24,:)'"/1 -> dotprod24/1
  dotprod24/1 -> Mux/24
  "IW{1,1}(25,:)'"/1 -> dotprod25/1
  dotprod25/1 -> Mux/25
  "IW{1,1}(26,:)'"/1 -> dotprod26/1
  dotprod26/1 -> Mux/26
  "IW{1,1}(27,:)'"/1 -> dotprod27/1
  dotprod27/1 -> Mux/27
  "IW{1,1}(28,:)'"/1 -> dotprod28/1
  dotprod28/1 -> Mux/28
  "IW{1,1}(29,:)'"/1 -> dotprod29/1
  dotprod29/1 -> Mux/29
  "IW{1,1}(30,:)'"/1 -> dotprod30/1
  dotprod30/1 -> Mux/30
  Mux/1 -> "iz{1,1}"/1

== system robotarm_part_both/NN_cex_1/Layer 2/Delays 1 ==
  "p{2}" : Inport  PortDimensions=30
      mask Display: e = 0.06;c1 = [120 230 180]/255;c2 = ([120 230 180]+0)/(256+128);c3 = ([120 230 180]+128)/(256+128);patch([0 1 1 0],[0 0 1 1],c1);patch([0 1 1 1-e 1-e 0+e],[0 0 1 1-e 0+e 0+e],c2);patch([0 0 1 1-e 0+e 0+e],[0 1 1 1-e 1-e 0+e],c3);plot([0 1 1 0 0],[0 0 1 1 0]);
  mux : Mux  Inputs=1
      mask Display: e = 0.06;c1 = [120 150 230]/255;c2 = ([120 150 230]+0)/383;c3 = ([120 150 230]+128)/383;patch([0 1 1 0],[0 0 1 1],c1);patch([0 1 1 1-e 1-e 0+e],[0 0 1 1-e 0+e 0+e],c2);patch([0 0 1 1-e 0+e 0+e],[0 1 1 1-e 1-e 0+e],c3);plot([0 1 1 0 0],[0 0 1 1 0]);disp('Mux')
  "pd{2,1}" : Outport
      mask Display: e = 0.06;c1 = [120 230 180]/255;c2 = ([120 230 180]+0)/(256+128);c3 = ([120 230 180]+128)/(256+128);patch([0 1 1 0],[0 0 1 1],c1);patch([0 1 1 1-e 1-e 0+e],[0 0 1 1-e 0+e 0+e],c2);patch([0 0 1 1-e 0+e 0+e],[0 1 1 1-e 1-e 0+e],c3);plot([0 1 1 0 0],[0 0 1 1 0]);
  wires:
  "p{2}"/1 -> mux/1
  mux/1 -> "pd{2,1}"/1
